simulink model "MicrowaveOven"  (R2020a)
settings: Solver=VariableStepAuto  StartTime=0.0  StopTime=500  RelTol=1e-3
settings Model: EnablePacing=on  Creator=jatin  LastModifiedBy=jatin

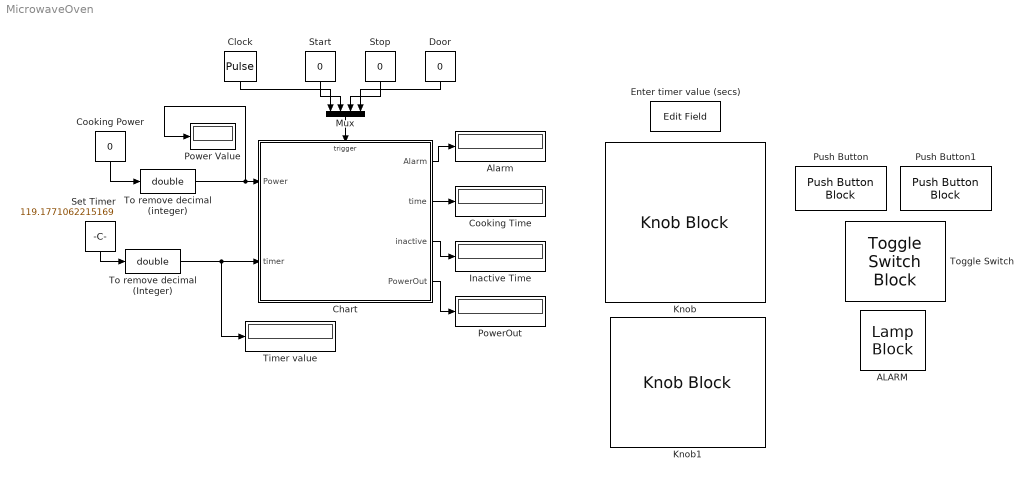
== system MicrowaveOven ==
  ALARM : LampBlock
  Alarm : Display
  Chart : Stateflow chart  TreatAsAtomicUnit=on
  Clock : DiscretePulseGenerator  PulseType=Time based  Period=1  PulseWidth=50
  Cooking Power : Constant  Value=0  OutDataTypeStr=uint32
  Cooking Time : Display
  Door : Constant  Value=0
  Enter timer value (secs) : EditField  Tag=Enter timer value  LabelPosition=Hide  ShowInitialText=on  Alignment=Center
  Inactive Time : Display
  Knob : KnobBlock  ScaleMax=1000  TickInterval=100
  Knob1 : KnobBlock  ScaleMax=800  TickInterval=100
  Mux : Mux
  Power Value : Display
  PowerOut : Display
  Push Button : PushButtonBlock  ButtonText=Start
  Push Button1 : PushButtonBlock  ButtonText=Stop
  Set Timer : Constant  Value=119.1771062215169  OutDataTypeStr=uint32
  Start : Constant  Value=0
  Stop : Constant  Value=0
  Timer value : Display
  To remove decimal (Integer) : DataTypeConversion  OutDataTypeStr=double
  To remove decimal (integer) : DataTypeConversion  OutDataTypeStr=double
  Toggle Switch : ToggleSwitchBlock  LabelPosition=Hide
      settings: Values={{'Close Door', 'Open Door'}, [0 1]}
  wires:
  Mux/1 -> Chart/Trigger
  Clock/1 -> Mux/1
  Start/1 -> Mux/2
  Stop/1 -> Mux/3
  Door/1 -> Mux/4
  Cooking Power/1 -> To remove decimal (integer)/1
  Chart/1(Alarm) -> Alarm/1
  Chart/2(time) -> Cooking Time/1
  Chart/3(inactive) -> Inactive Time/1
  Set Timer/1 -> To remove decimal (Integer)/1
  To remove decimal (Integer)/1 -> Timer value/1, Chart/2(timer)
  To remove decimal (integer)/1 -> Chart/1(Power), Power Value/1
  Chart/4(PowerOut) -> PowerOut/1

== stateflow chart MicrowaveOven/Chart ==
  settings: executeAtInitialization=1
  state TimeState
    time = timer;T= timer;
    PowerOut=Power;
    en: inactive=0;
    on TIC: inactive_time();
  state CookingState
    Alarm=0;
    newT= timer;
    on TIC: decrease_time();
  state IdleState
    en: time=0;
    du: PowerOut=Power;
  state StopState
    en: reset=1; inactive=0;
    on TIC: inactive_time();
  state Door
    reset=1;
  state InactiveTime
    en: inactive=0;
    on TIC: inactive_time();
  state DoorState
    reset=1;
  StopState -> IdleState [order 3] : [time==0]
  StopState -> IdleState [order 1] : stop/{time=0;}
  CookingState -> IdleState [order 3] : [reset == 1]{Alarm=1;}
  StopState -> CookingState [order 2] : start/{reset=0;}
  (default) -> IdleState
  IdleState -> TimeState [order 2] : [hasChanged(timer)==1]
  TimeState -> CookingState [order 1] : start/{reset=0;}
  TimeState -> IdleState [order 2] : [time==0]
  CookingState -> StopState [order 2] : stop
  IdleState -> DoorState [order 1] : door
  CookingState -> Door [order 1] : door
  StopState -> Door [order 4] : door
  Door -> StopState : door
  TimeState -> DoorState [order 3] : door
  DoorState -> TimeState : door
  data: reset local; Power input; Alarm output; newT local; T local; timer input; time output; inactive output; PowerOut output
  events: TIC input RISING_EDGE_EVENT; start input RISING_EDGE_EVENT; stop input RISING_EDGE_EVENT; door input EITHER_EDGE_EVENT
  function decrease_time:
    | function decrease_time
    | if newT == T
    |     if reset == 0
    |         time = time-1;
    |         if time<=0
    |             reset = 1;
    |         end
    |     end
    | else T=newT;
    |     time = newT;
    | end
  function inactive_time:
    | function inactive_time
    | inactive = inactive+1;
    | if inactive>=10
    |     time=0;
    |     inactive = 0;
    | end
    | if hasChanged(timer)
    |     inactive=0;
    | end
